simulink model "Digital"  (R2022b)
settings: Solver=VariableStepAuto  StartTime=0.0  StopTime=10.0  RelTol=1e-3
libraries: vivadosimlib x1
settings Model: Creator=Ali-Laptop  LastModifiedBy=Ali-Laptop

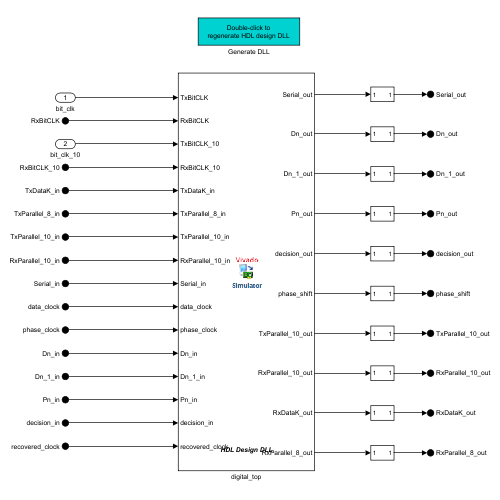
[thumbnail: Simulink's stored preview of the top-level diagram]
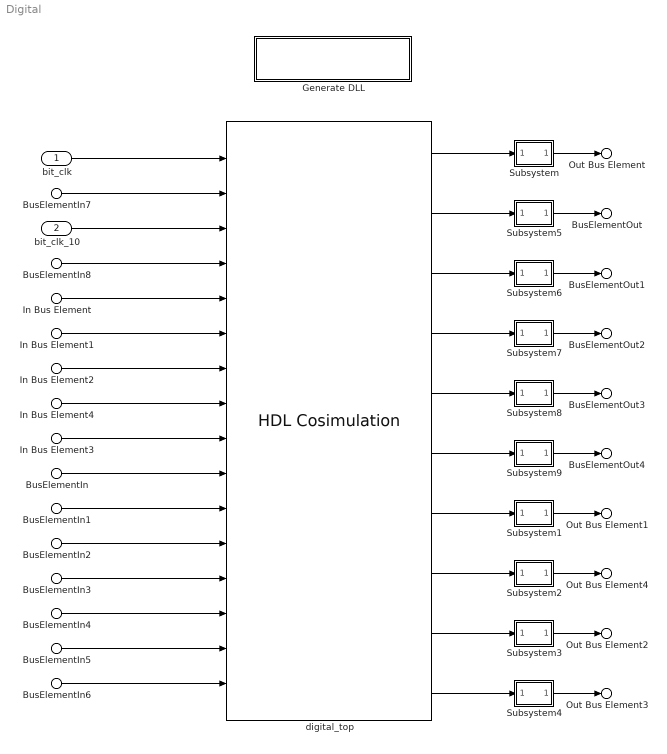
== system Digital ==
  bit_clk : Inport
  bit_clk_10 : Inport  Port=2
  In Bus Element : Inport  Port=3  PortName=tx_in  Element=TxDataK_in
  In Bus Element1 : Inport  Port=3  PortName=tx_in  Element=TxParallel_8_in
  In Bus Element2 : Inport  Port=3  PortName=tx_in  Element=TxParallel_10_in
  BusElementIn7 : Inport  Port=4  PortName=rx_in  Element=RxBitCLK
  BusElementIn8 : Inport  Port=4  PortName=rx_in  Element=RxBitCLK_10
  In Bus Element3 : Inport  Port=4  PortName=rx_in  Element=Serial_in
  In Bus Element4 : Inport  Port=4  PortName=rx_in  Element=RxParallel_10_in
  BusElementIn : Inport  Port=4  PortName=rx_in  Element=data_clock
  BusElementIn1 : Inport  Port=4  PortName=rx_in  Element=phase_clock
  BusElementIn2 : Inport  Port=4  PortName=rx_in  Element=Dn_in
  BusElementIn3 : Inport  Port=4  PortName=rx_in  Element=Dn_1_in
  BusElementIn4 : Inport  Port=4  PortName=rx_in  Element=Pn_in
  BusElementIn5 : Inport  Port=4  PortName=rx_in  Element=decision_in
  BusElementIn6 : Inport  Port=4  PortName=rx_in  Element=recovered_clock
  Generate DLL : Subsystem
      settings: OpenFcn=eval('hdlverifier_gendll_digital_top');
      mask Display: disp(['Double-click to' char(10) 'regenerate HDL design DLL'])
  Subsystem : Subsystem
  Subsystem1 : Subsystem
  Subsystem2 : Subsystem
  Subsystem3 : Subsystem
  Subsystem4 : Subsystem
  Subsystem5 : Subsystem
  Subsystem6 : Subsystem
  Subsystem7 : Subsystem
  Subsystem8 : Subsystem
  Subsystem9 : Subsystem
  digital_top : vivadosimlib/HDL Cosimulation  PortPaths=/digital_top/TxBitCLK;/digital_top/RxBitCLK;/digital_top/TxBitCLK_10;/digital_top/RxBitCLK_10;/digital_top/TxDataK_in;/digital_top/TxParallel_8_in;/digital_top/TxParallel_10_in;/digital_top/RxParallel_10_in;/digital_top/Serial_in;/digital_top/data_clock;/digital_top/phase_clock;/digital_top/Dn_in;/digital_top/Dn_1_in;/digital_top/Pn_in;/digital_top/decision_in;/digital_top/recovered_clock;/digital_top/Serial_out;/digital_top/Dn_out;/digital_top/Dn_1_out;/digital_top/Pn_out;/digital_top/decision_out;/digital_top/phase_shift;/digital_top/TxParallel_10_out;/digital_top/RxParallel_10_out;/digital_top/RxDataK_out;/digital_top/RxParallel_8_out;  PortModes=[1 1 1 1 1 1 1 1 1 1 1 1 1 1 1 1 2 2 2 2 2 2 2 2 2 2 ]  PortTimes=[-1,-1,-1,-1,-1,-1,-1,-1,-1,-1,-1,-1,-1,-1,-1,-1,-1,-1,-1,-1,-1,-1,-1,-1,-1,-1]  PortSigns=[-1,-1,-1,-1,-1,-1,-1,-1,-1,-1,-1,-1,-1,-1,-1,-1,-1,-1,-1,-1,-1,-1,-1,-1,-1,-1,]  PortFracLengths=[0,0,0,0,0,0,0,0,0,0,0,0,0,0,0,0,0,0,0,0,0,0,0,0,0,0]  CommLocal=on  CommSharedMemory=off  CommPortNumber=0  CommShowInfo=on  ClockPaths=/digital_top/Reset;  ClockModes=[4 ]  ClockTimes=[8e-12 ]  TclPreSimCommand="puts \"Running Simulink Cosimulation block.\""  TclPostSimCommand="puts \"done\""  TimingMode=s  TimingScaleFactor=1  idxCellArray={'UNUSED_VAR'}  CosimBypass=Full Simulation  AllowDirectFeedthrough=on  ProductName=EDA Simulator Link VS  RunAutoTimescale=off  HdlClocks=0  PreRunTime=8  PreRunTimeUnit=ps
  Out Bus Element : Outport  PortName=tx_out  Element=Serial_out
  Out Bus Element1 : Outport  PortName=tx_out  Element=TxParallel_10_out
  Out Bus Element2 : Outport  Port=2  PortName=rx_out  Element=RxDataK_out
  Out Bus Element3 : Outport  Port=2  PortName=rx_out  Element=RxParallel_8_out
  Out Bus Element4 : Outport  Port=2  PortName=rx_out  Element=RxParallel_10_out
  BusElementOut : Outport  Port=2  PortName=rx_out  Element=Dn_out
  BusElementOut1 : Outport  Port=2  PortName=rx_out  Element=Dn_1_out
  BusElementOut2 : Outport  Port=2  PortName=rx_out  Element=Pn_out
  BusElementOut3 : Outport  Port=2  PortName=rx_out  Element=decision_out
  BusElementOut4 : Outport  Port=2  PortName=rx_out  Element=phase_shift
  wires:
  bit_clk_10/1 -> digital_top/3
  bit_clk/1 -> digital_top/1
  digital_top/1 -> Subsystem/1(In1)
  digital_top/7 -> Subsystem1/1(In1)
  Subsystem2/1(Out1) -> Out Bus Element4/1
  digital_top/8 -> Subsystem2/1(In1)
  digital_top/10 -> Subsystem4/1(In1)
  digital_top/9 -> Subsystem3/1(In1)
  Subsystem3/1(Out1) -> Out Bus Element2/1
  Subsystem4/1(Out1) -> Out Bus Element3/1
  Subsystem/1(1) -> Out Bus Element/1
  Subsystem1/1(1) -> Out Bus Element1/1
  In Bus Element/1 -> digital_top/5
  In Bus Element1/1 -> digital_top/6
  In Bus Element2/1 -> digital_top/7
  In Bus Element4/1 -> digital_top/8
  In Bus Element3/1 -> digital_top/9
  BusElementIn/1 -> digital_top/10
  BusElementIn1/1 -> digital_top/11
  BusElementIn2/1 -> digital_top/12
  BusElementIn3/1 -> digital_top/13
  BusElementIn4/1 -> digital_top/14
  BusElementIn5/1 -> digital_top/15
  BusElementIn6/1 -> digital_top/16
  Subsystem5/1(1) -> BusElementOut/1
  digital_top/2 -> Subsystem5/1(In1)
  Subsystem6/1(1) -> BusElementOut1/1
  digital_top/3 -> Subsystem6/1(In1)
  Subsystem7/1(1) -> BusElementOut2/1
  digital_top/4 -> Subsystem7/1(In1)
  Subsystem8/1(1) -> BusElementOut3/1
  digital_top/5 -> Subsystem8/1(In1)
  Subsystem9/1(1) -> BusElementOut4/1
  digital_top/6 -> Subsystem9/1(In1)
  BusElementIn7/1 -> digital_top/2
  BusElementIn8/1 -> digital_top/4

== system Digital/Generate DLL ==

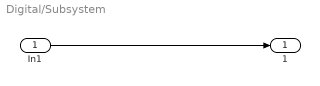
== system Digital/Subsystem ==
  In1 : Inport
  1 : Outport  SampleTime=1e-10
  wires:
  In1/1 -> 1/1

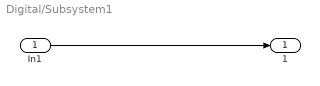
== system Digital/Subsystem1 ==
  In1 : Inport
  1 : Outport  SampleTime=1e-10
  wires:
  In1/1 -> 1/1

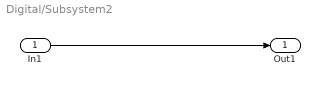
== system Digital/Subsystem2 ==
  In1 : Inport
  Out1 : Outport  SampleTime=1e-10
  wires:
  In1/1 -> Out1/1

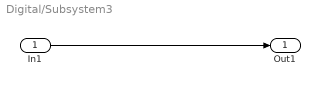
== system Digital/Subsystem3 ==
  In1 : Inport
  Out1 : Outport  SampleTime=1e-10
  wires:
  In1/1 -> Out1/1

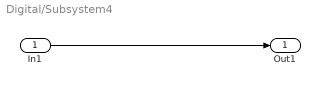
== system Digital/Subsystem4 ==
  In1 : Inport
  Out1 : Outport  SampleTime=1e-10
  wires:
  In1/1 -> Out1/1

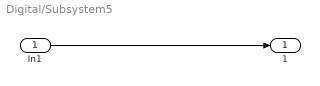
== system Digital/Subsystem5 ==
  In1 : Inport
  1 : Outport  SampleTime=1e-10
  wires:
  In1/1 -> 1/1

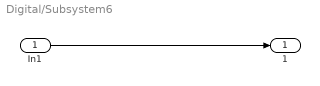
== system Digital/Subsystem6 ==
  In1 : Inport
  1 : Outport  SampleTime=1e-10
  wires:
  In1/1 -> 1/1

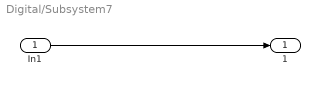
== system Digital/Subsystem7 ==
  In1 : Inport
  1 : Outport  SampleTime=1e-10
  wires:
  In1/1 -> 1/1

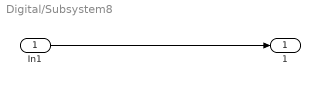
== system Digital/Subsystem8 ==
  In1 : Inport
  1 : Outport  SampleTime=1e-10
  wires:
  In1/1 -> 1/1

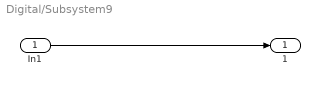
== system Digital/Subsystem9 ==
  In1 : Inport
  1 : Outport  SampleTime=1e-10
  wires:
  In1/1 -> 1/1
